simulink subsystem "newtonianMechanics"  (R2026a)
settings: Solver=VariableStepAuto
undefined symbols (not defined in the file): aero, Fx, fz_linspace, kappa
settings Model: Creator=lholliday  LastModifiedBy=lholliday

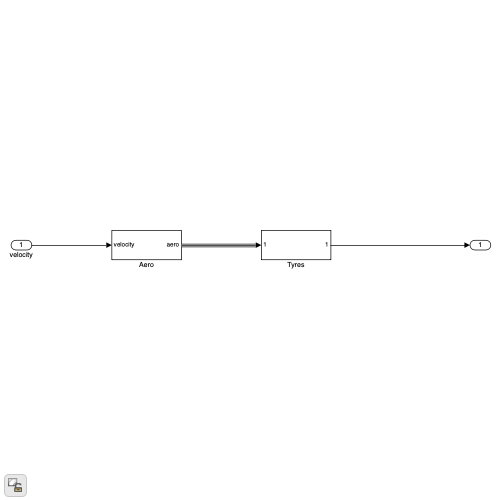
[thumbnail: Simulink's stored preview of the top-level diagram]
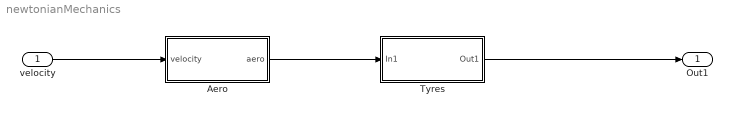
== system newtonianMechanics ==
  velocity : Inport
  Aero : Subsystem
  Tyres : Subsystem
  Out1 : Outport
  wires:
  Tyres/1(Out1) -> Out1/1
  velocity/1 -> Aero/1(velocity)
  Aero/1(aero) -> Tyres/1(In1)

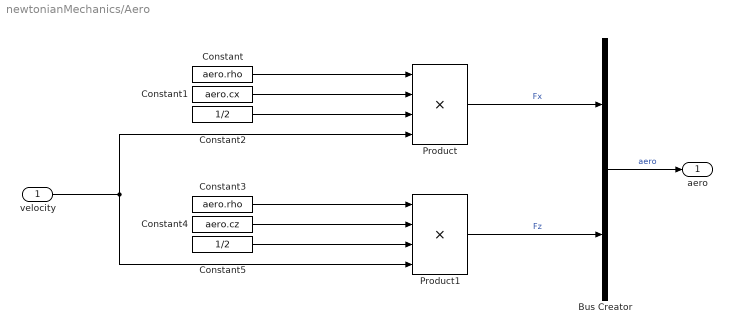
== system newtonianMechanics/Aero ==
  velocity : Inport
  Bus Creator : BusCreator  Inputs=2
  Constant : Constant  Value=aero.rho
  Constant1 : Constant  Value=aero.cx
  Constant2 : Constant  Value=1/2
  Constant3 : Constant  Value=aero.rho
  Constant4 : Constant  Value=aero.cz
  Constant5 : Constant  Value=1/2
  Product : Product  Inputs=4
  Product1 : Product  Inputs=4
  aero : Outport
  wires:
  Constant4/1 -> Product1/2
  Constant3/1 -> Product1/1
  velocity/1 -> Product1/4, Product/4
  Constant5/1 -> Product1/3
  Constant1/1 -> Product/2
  Constant2/1 -> Product/3
  Constant/1 -> Product/1
  Product/1 -> Bus Creator/1  "Fx"
  Bus Creator/1 -> aero/1  "aero"
  Product1/1 -> Bus Creator/2  "Fz"

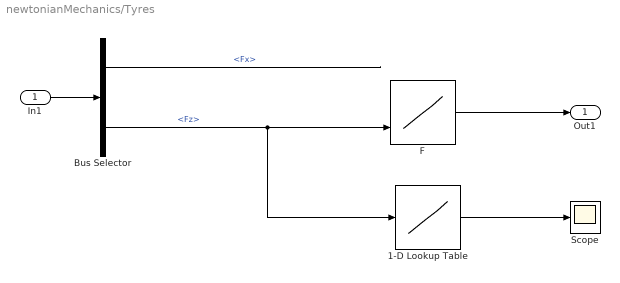
== system newtonianMechanics/Tyres ==
  In1 : Inport
  1-D Lookup Table : Lookup_n-D  NumberOfTableDimensions=1  BreakpointsForDimension1=fz_linspace  Table=Fx(100,:)  InternalRulePriority=Speed  RndMeth=Simplest
  Bus Selector : BusSelector  OutputSignals=Fx,Fz
  F : Lookup_n-D  LookupTableObject=fx_basic_LUT  BreakpointsForDimension1=kappa  BreakpointsForDimension2=fz_linspace  Table=Fx  InternalRulePriority=Speed  RndMeth=Simplest
      settings: InputPortMap=u0,u1
  Scope : Scope
      settings: ActiveDisplayYMinimum=-2899.3859124150231  ActiveDisplayYMaximum=-2894.37009706589  DataLoggingVariableName=ScopeData9
  Out1 : Outport
  wires:
  1-D Lookup Table/1 -> Scope/1
  F/1 -> Out1/1
  Bus Selector/2 -> F/2, 1-D Lookup Table/1  "<Fz>"
  Bus Selector/1 -> ?  "<Fx>"
  In1/1 -> Bus Selector/1
